simulink model "eclipse_target_2"  (Simulink 8.3)
settings: Solver=FixedStepDiscrete  StartTime=0.0  StopTime=inf  FixedStep=Ts  RelTol=1e-3
PreLoadFcn:
  | load_waypoints
libraries: idelinklib_tgtpref x1, instrumentlib x1
settings Model: Creator=janosch  LastModifiedBy=lucas  SimulationMode=external
settings DataIOCC: LimitDataPoints=off  SaveOutput=off  SaveTime=off
settings OptimizationCC: ExpressionDepthLimit=2147483647  OptimizeModelRefInitCode=on  LifeSpan=1
settings DebuggingCC: ParameterPrecisionLossMsg=none  FcnCallInpInsideContextMsg=UseLocalSettings
settings HardwareCC: ProdIntDivRoundTo=Zero  ProdEndianess=LittleEndian  ProdHWDeviceType=Intel Pentium
settings RTWCC: SystemTargetFile=idelink_ert.tlc  GenerateMakefile=off  TemplateMakefile=idelink_ert.tmf  Description=Embedded IDE Link ERT  ProcessScript=idelink_ert_make_rtw_hook
settings CodeAppCC: IgnoreCustomStorageClasses=off  CustomSymbolStrType=$N$R$M  InternalIdentifier=Classic
settings ERTFactory: TargetFcnLib=ansi_tfl_table_tmw.mat  GenFloatMathFcnCalls=NOT IN USE  TargetLangStandard=C89/C90 (ANSI)  CodeReplacementLibrary=None  UtilityFuncGeneration=Auto  ERTMultiwordTypeDef=System defined  ERTMultiwordLength=256  MultiwordLength=2048  GenerateFullHeader=on  GenerateSampleERTMain=off  GenerateTestInterfaces=off  ModelReferenceCompliant=on  ParMdlRefBuildCompliant=off  CompOptLevelCompliant=off  ConcurrentExecutionCompliant=on  IncludeMdlTerminateFcn=on  GeneratePreprocessorConditionals=Disable all  CombineOutputUpdateFcns=on  CombineSignalStateStructs=off  SuppressErrorStatus=off  ERTFirstTimeCompliant=off  IncludeFileDelimiter=Auto  ERTCustomFileBanners=on  SupportAbsoluteTime=on  LogVarNameModifier=rt_  MatFileLogging=off  MultiInstanceERTCode=off  CodeInterfacePackaging=Nonreusable function  SupportNonFinite=on  SupportComplex=on  PurelyIntegerCode=off  SupportContinuousTime=off  SupportNonInlinedSFcns=on  SupportVariableSizeSignals=off  EnableShiftOperators=on  ParenthesesLevel=Nominal  MATLABClassNameForMDSCustomization=linkfoundation.pjtgenerator.IdelinkCustomization  ModelStepFunctionPrototypeControlCompliant=on  CPPClassGenCompliant=off  AutosarCompliant=off  GRTInterface=off  GenerateAllocFcn=off  GenerateASAP2=off  ExtMode=on  ExtModeTransport=0  ExtModeStaticAlloc=off  ExtModeStaticAllocSize=1000000  ExtModeTesting=off  ExtModeMexFile=ext_comm  ExtModeIntrfLevel=Level1  InlinedParameterPlacement=Hierarchical  TargetOS=BareBoardExample  MultiInstanceErrorCode=Error  RateGroupingCode=on  RootIOFormat=Individual arguments  RTWCAPISignals=off  RTWCAPIParams=off  RTWCAPIStates=off  RTWCAPIRootIO=off  ERTSrcFileBannerTemplate=ert_code_template.cgt  ERTHdrFileBannerTemplate=ert_code_template.cgt  ERTDataSrcFileTemplate=ert_code_template.cgt  ERTDataHdrFileTemplate=ert_code_template.cgt  ERTCustomFileTemplate=example_file_process.tlc  EnableDataOwnership=off  SignalDisplayLevel=10  ParamTuneLevel=10  GlobalDataDefinition=Auto  DataDefinitionFile=global.c  GlobalDataReference=Auto  ERTFilePackagingFormat=Modular  DataReferenceFile=global.h  PreserveExpressionOrder=off  PreserveIfCondition=off  ConvertIfToSwitch=off  PreserveExternInFcnDecls=on  SuppressUnreachableDefaultCases=off  IndentStyle=K&R  IndentSize=2  EnableUserReplacementTypes=off  MemSecPackage=--- None ---  MemSecDataConstants=Default  MemSecDataIO=Default  MemSecDataInternal=Default  MemSecDataParameters=Default  MemSecFuncInitTerm=Default  MemSecFuncExecute=Default  MemSecFuncSharedUtil=Default  AdaptorName=Eclipse  exportIDEObj=on  ideObjName=IDE_Obj  oldideObjName=IDE_Obj  ideObjTimeout=50  oldideObjTimeout=50  ideObjBuildTimeout=1000  oldideObjBuildTimeout=1000  TargetPrefTimeStamp=27-May-2014 00:17:19  ProfileGenCode=off  profileBy=Tasks  ProfileNumSamples=100  InlineDSPBlks=off  projectOptions=Custom  debugCompilerOptions="-g -D\"_DEBUG\""  releaseCompilerOptions=-O2  getCompilerOptions=off  resetCompilerOptions=off  debugLinkerOptions=-lm  releaseLinkerOptions=-lm  customLinkerOptions=-lm  linkerOptionsStr=-lm  getLinkerOptions=off  resetLinkerOptions=off  systemStackSize=512  systemHeapSize=512  buildFormat=Project  buildAction=Build  overrunNotificationMethod=None  overrunNotificationFcn=myfunction  oldoverrunNotificationFcn=myfunction  configurePIL=off  configPILBlockAction=Create_PIL_block_build_and_download  TargetResourceManagerActiveTab=0  DiagnosticActions=warning
settings ConfigurationSet: Description=SimMechanics 2G
settings TargetHardwareResources: Description=Target Hardware Resources Component
settings MATStruct: cache=[]  boardType=Custom  isSimulator=[0.0]  enableHSRTDX=[0.0]  versionNumber=2.9.1  enableDSPBIOSTab=[0.0]  RTOS=Linux  peripherals=[]  procName=4444  boardName=localhost  realtimesupport=off  tag=eclipseidetgtpref  deviceID=Intel x86/Pentium  subFamily=host  cpuClockRateMHz=[0.0]  codegenhookpoint=host  numSections=[19.0]  numRTOS=[3.0]  defaultSysStackSize=[512.0]  isBuiltIn=[1.0]  numBanks=[3.0]  numCacheLvl=[0.0]  name=sram_memory  contents=Code & Data  space=Internal  addr=[4194304.0]  size=[861226034.0]  isremovable=[0.0]  iscontentsfixed=[0.0]  createHeap=[0.0]  heapSize=[256.0]  defineLabel=[0.0]  heapLabel=segment_name  label=None  timer=[]  timerprescaler=[]  description=Program code  codeObjectMem=sram_memory  dataObjectMem=sram_memory  section=[]  enable=off  schedulerType=Rate priority  schedulingMode=real-time  baseRatePriority=[40.0]  stackSize=[4096.0]  staticStackMemSegment=sram_memory  dynamicStackMemSegment=sram_memory  errId=[]

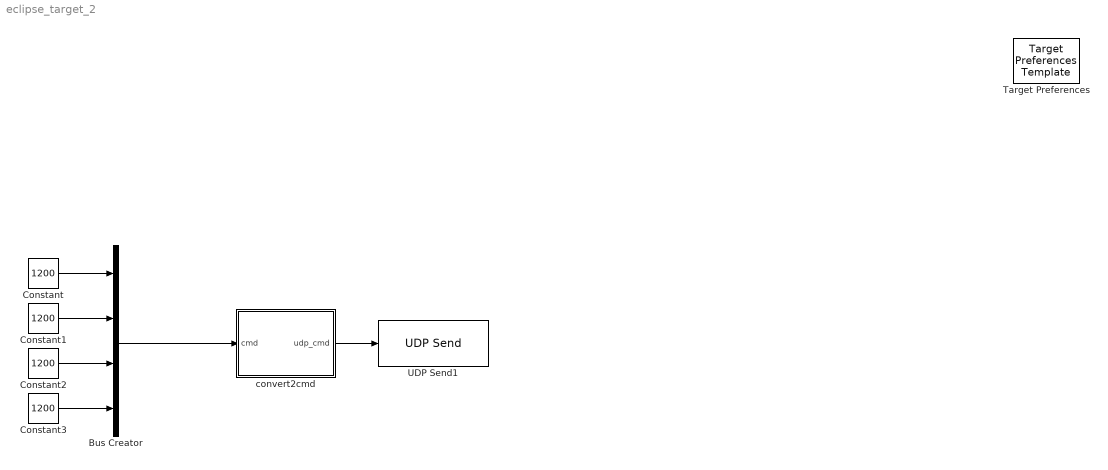
== system eclipse_target_2 ==
  Bus Creator : BusCreator
  Constant{,1..3} (4 alike) : Constant  Value=1200
  Target Preferences : idelinklib_tgtpref/Target Preferences Template  Tag=eclipseidetgtpref  library=off
  UDP Send1 : instrumentlib/UDP Send  Priority=2  Host=127.0.0.1  Port=51001  LocalPort=51000  EnableBlockingMode=on  ByteOrder=LittleEndian
  convert2cmd : Subsystem
  wires:
  convert2cmd/1(udp_cmd) -> UDP Send1/1
  Constant/1 -> Bus Creator/1
  Constant1/1 -> Bus Creator/2
  Constant2/1 -> Bus Creator/3
  Constant3/1 -> Bus Creator/4
  Bus Creator/1 -> convert2cmd/1(cmd)

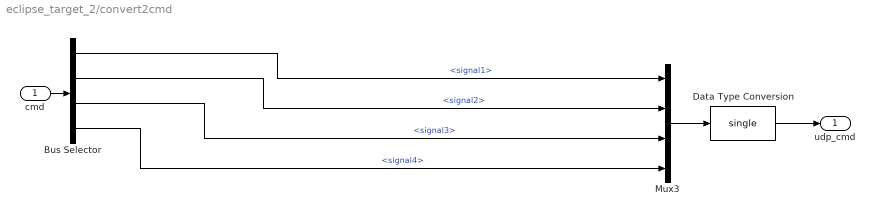
== system eclipse_target_2/convert2cmd ==
  cmd : Inport
  Bus Selector : BusSelector  OutputSignals=signal1,signal2,signal3,signal4
  Data Type Conversion : DataTypeConversion  OutDataTypeStr=single
  Mux3 : Mux
  udp_cmd : Outport
  wires:
  Bus Selector/4 -> Mux3/4  "<signal4>"
  Bus Selector/2 -> Mux3/2  "<signal2>"
  Bus Selector/1 -> Mux3/1  "<signal1>"
  cmd/1 -> Bus Selector/1
  Data Type Conversion/1 -> udp_cmd/1
  Mux3/1 -> Data Type Conversion/1
  Bus Selector/3 -> Mux3/3  "<signal3>"
